simulink model "MinSegNano_Demo"  (R2015a)
settings: Solver=FixedStepDiscrete  StartTime=0.0  StopTime=inf  FixedStep=.01  RelTol=1e-3
libraries: RASPlib x9, arduinolib x4, MinSegLibrary_MinSegNano x2
settings Model: ExtModeTrigDuration=2  Creator=Alec  LastModifiedBy=hurstj
settings OptimizationCC: ExpressionDepthLimit=2147483647  OptimizeModelRefInitCode=on  LifeSpan=1
settings DebuggingCC: UnderspecifiedInitializationDetection=Classic  MergeDetectMultiDrivingBlocksExec=none  StateNameClashWarn=warning
settings HardwareCC: ProdBitPerInt=16  ProdBitPerPointer=8  ProdIntDivRoundTo=Zero  ProdEndianess=LittleEndian  ProdWordSize=8  ProdHWDeviceType=Atmel->AVR
settings RTWCC: SystemTargetFile=realtime.tlc  GenerateMakefile=off  TemplateMakefile=realtime.tmf  Description=Real-Time Toolbox  RTWVerbose=off
settings CodeAppCC: CustomSymbolStrType=$N$R$M  InternalIdentifier=Classic
settings ERTTargetCC: CombineOutputUpdateFcns=off  ExtModeTransport=3  ExtModeMexArgs=0 1 9600  ERTSrcFileBannerTemplate=realtime_code_template.cgt  ERTHdrFileBannerTemplate=realtime_code_template.cgt  ERTDataSrcFileTemplate=realtime_code_template.cgt  ERTDataHdrFileTemplate=realtime_code_template.cgt  ERTCustomFileTemplate=realtime_file_process.tlc

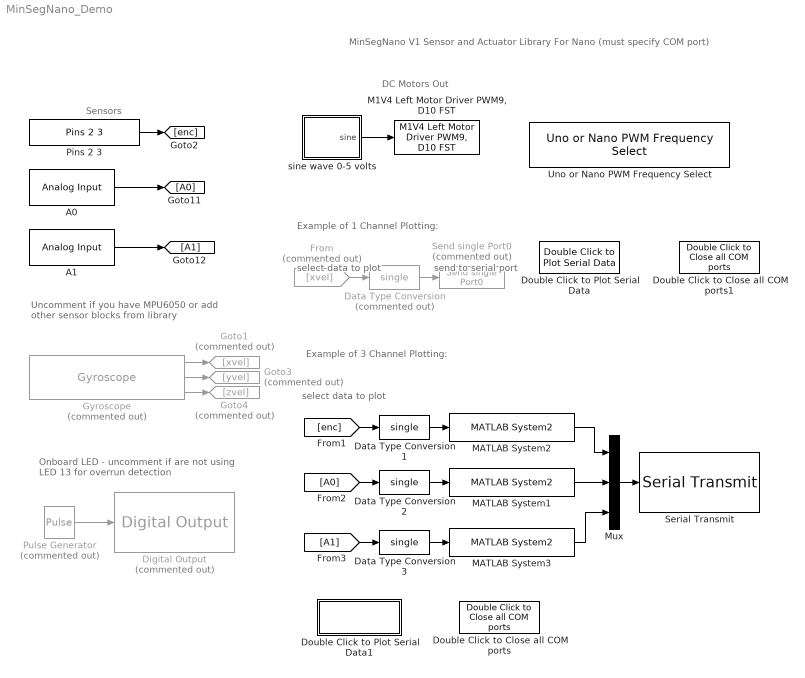
== system MinSegNano_Demo ==
  note: Onboard LED - uncomment if are not
      | using LED 13 for overrun detection
  note: Uncomment if you have MPU6050 or
      | add other sensor blocks from library
  note: Example of 1 Channel Plotting:
  note: send to serial port
  note: select data to plot
  note: DC Motors Out
  note: Sensors
  note: MinSegNano V1 Sensor and Actuator Library
      | For Nano (must specify COM port)
  note: Example of 3 Channel Plotting:
  note: select data to plot
  A0 : arduinolib/Analog Input  pinNumber=0  sampleTime=-1  blockPlatform=arduino
  A1 : arduinolib/Analog Input  pinNumber=1  sampleTime=-1  blockPlatform=arduino
  Data Type Conversion : DataTypeConversion  Commented=on  OutDataTypeStr=single
  Data Type Conversion1 : DataTypeConversion  OutDataTypeStr=single
  Data Type Conversion2 : DataTypeConversion  OutDataTypeStr=single
  Data Type Conversion3 : DataTypeConversion  OutDataTypeStr=single
  Digital Output : arduinolib/Digital Output  Commented=on  pinNumber=13  blockPlatform=arduino
  Double Click to Close all COM ports : RASPlib/Double Click to Close all COM ports
  Double Click to Close all COM ports1 : RASPlib/Double Click to Close all COM ports
  Double Click to Plot Serial Data : RASPlib/Double Click to Plot Serial Data  COMport=28  BaudRate=9600  NumSamples=500  DataType=single  Ncx=1
  Double Click to Plot Serial Data1 : Subsystem  mask{COMport=28, BaudRate=9600, NumSamples=500, DataType=single, Ncx=3}
      mask prompts: COMport "COM Port:"; BaudRate "Baud Rate (needs to be same as Baud Rate in configuration parameters)"; NumSamples "Number of samples to plot"; DataType "Data Type of data being sent"; Ncx "N - Number of muxed channels"
      mask TypeOptions DataType: uint8 | int16 | single
      mask DialogControl DescTextVar Prompt: Plot single channel data received from the serial line.  View Matlab command window for connection and plot information.  After stopping graph, the data is stored in the variables fdat and wdat in the workspace.  Both variables are also saved to the file fdat.mat in the current directory.  This block does not download any code to the hardware - just a block to plot data recieved. The ploting procedure can be modified by editing the file SerialPlot.m.
      mask DialogControl Control3 Prompt: text here
      mask DialogControl Control2 Prompt: Click Here to Plot Data
      mask DialogControl Control2 Callback: SerialPlot(['COM' get_param(gcb,'COMport')], get_param(gcb,'DataType'), str2num(get_param(gcb,'NumSamples')), str2num(get_param(gcb,'BaudRate')),str2num(get_param(gcb,'Ncx')))
      mask Display: disp('SerialPlot')
  From : From  Commented=on  GotoTag=xvel
  Goto1 : Goto  Commented=on  GotoTag=xvel
  Goto3 : Goto  Commented=on  GotoTag=yvel
  Goto4 : Goto  Commented=on  GotoTag=zvel
  Gyroscope : RASPlib/Gyroscope  Commented=on  DLPFmode=0
  "M1V4 Left Motor Driver PWM9, D10 FST" : MinSegLibrary_MinSegNano/M1V4 Left Motor Driver PWM9, D10 FST  Vsupply=3.25
  MATLAB System1 : RASPlib/Send single Port0/MATLAB System2  SimulateUsing=Code generation
  MATLAB System2 : RASPlib/Send single Port0/MATLAB System2  SimulateUsing=Code generation
  MATLAB System3 : RASPlib/Send single Port0/MATLAB System2  SimulateUsing=Code generation
  Mux : Mux  Inputs=3
  Pins 2 3 : MinSegLibrary_MinSegNano/Pins 2 3  Encoder=0  PinA=2  PinB=3
  Pulse Generator : DiscretePulseGenerator  Commented=on  PulseType=Time based  Period=10  PulseWidth=5
  Send single Port0 : RASPlib/Send single Port0  Commented=on
  Serial Transmit : arduinolib/Serial Transmit  portNumber=0  blockPlatform=arduino
  Uno or Nano PWM Frequency Select : RASPlib/Uno or Nano PWM Frequency Select  Frequency=490Hz  Timer=1 - pins 9, 10
  sine wave 0-5 volts : Subsystem
  wires:
  sine wave 0-5 volts/1(sine) -> "M1V4 Left Motor Driver PWM9, D10 FST"/1
  A0/1 -> [A0]
  A1/1 -> [A1]
  Pins 2 3/1 -> [enc]
  From/1 -> Data Type Conversion/1
  Data Type Conversion/1 -> Send single Port0/1
  Gyroscope/1 -> Goto1/1
  MATLAB System1/1 -> Mux/2
  MATLAB System2/1 -> Mux/1
  [enc] -> Data Type Conversion1/1
  Data Type Conversion1/1 -> MATLAB System2/1
  [A0] -> Data Type Conversion2/1
  Data Type Conversion2/1 -> MATLAB System1/1
  Mux/1 -> Serial Transmit/1
  Data Type Conversion3/1 -> MATLAB System3/1
  MATLAB System3/1 -> Mux/3
  [A1] -> Data Type Conversion3/1
  Pulse Generator/1 -> Digital Output/1
  Gyroscope/2 -> Goto3/1
  Gyroscope/3 -> Goto4/1

== system MinSegNano_Demo/Double Click to Plot Serial Data1 ==

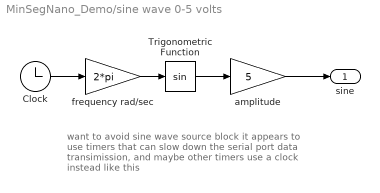
== system MinSegNano_Demo/sine wave 0-5 volts ==
  note: want to avoid sine wave source block
      | it appears to use timers that can slow down the
      | serial port data transimission, and maybe
      | other timers
      |
      | use a clock instead like this
  Clock : Clock
  Trigonometric Function : Trigonometry
  amplitude : Gain  Gain=5
  frequency rad/sec : Gain  Gain=2*pi
  sine : Outport
  wires:
  Clock/1 -> frequency rad/sec/1
  Trigonometric Function/1 -> amplitude/1
  frequency rad/sec/1 -> Trigonometric Function/1
  amplitude/1 -> sine/1
